simulink model "b747_lateral_openloop"  (R2025a)
settings: Solver=VariableStepAuto  StartTime=0.0  StopTime=T_end  RelTol=1e-3
undefined symbols (not defined in the file): A, B, C, D, T_end
libraries: simulink_extras x12
settings Model: Creator=User  LastModifiedBy=User

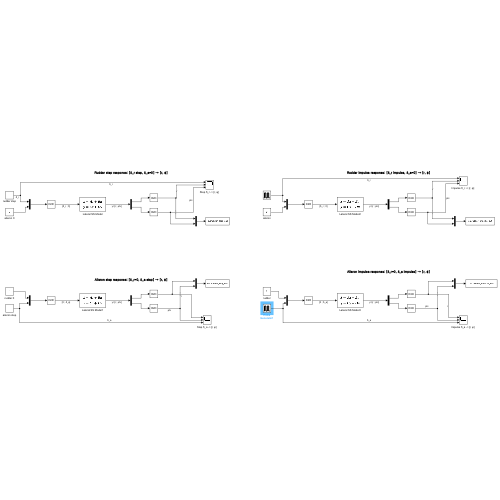
[thumbnail: Simulink's stored preview of the top-level diagram]
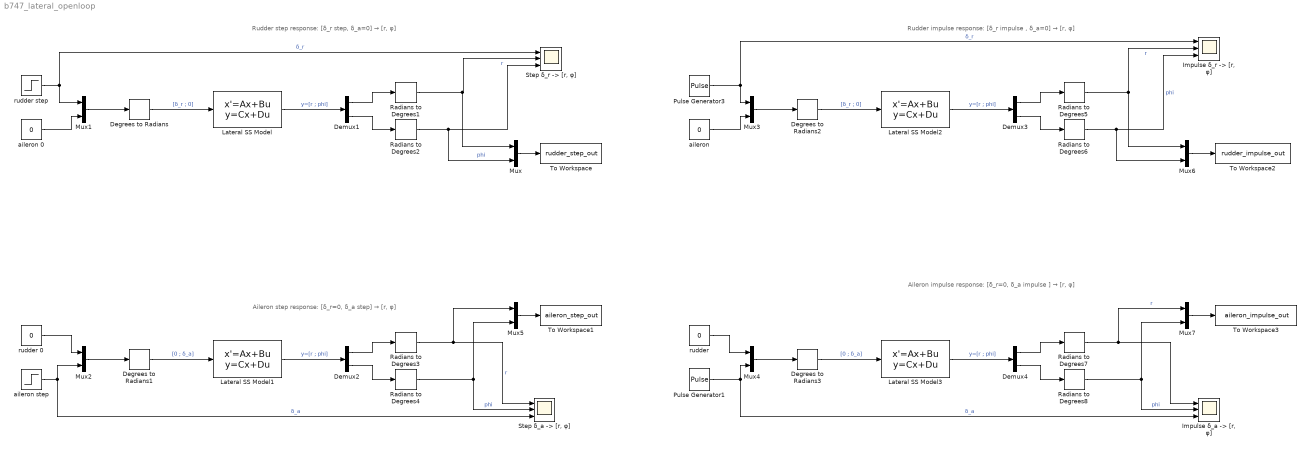
== system b747_lateral_openloop ==
  note: Rudder step response: [δ_r step, δ_a=0] → [r, φ]
  note: Aileron step response: [δ_r=0, δ_a step] → [r, φ]
  note: Aileron impulse response: [δ_r=0, δ_a impulse ] → [r, φ]
  note: Rudder impulse response: [δ_r impulse , δ_a=0] → [r, φ]
  Degrees to Radians{,1..3} (4 alike) : simulink_extras/Transformations/Degrees to Radians
  Demux{1..4} (4 alike) : Demux  Outputs=2
  "Impulse δ_a -> [r, φ] " : Scope  NumInputPorts=3
      settings: ActiveDisplayYMinimum=-7.0438793866264691  ActiveDisplayYMaximum=8.3524253239739448  DataLoggingVariableName=ScopeData6
  "Impulse δ_r -> [r, φ] " : Scope  NumInputPorts=3
      settings: ActiveDisplayYMinimum=-206.46074669660285  ActiveDisplayYMaximum=229.7370843531925  DataLoggingVariableName=ScopeData4
  Lateral SS Model{,1..3} (4 alike) : StateSpace  A=A  B=B  C=C  D=D  InitialCondition=0
  Mux{,1..7} (8 alike) : Mux  Inputs=2
  Pulse Generator1 : DiscretePulseGenerator  PulseType=Time based  Amplitude=20  Period=T_end  PulseWidth=0.125  PhaseDelay=1
  Pulse Generator3 : DiscretePulseGenerator  PulseType=Time based  Amplitude=20  Period=T_end  PulseWidth=0.125  PhaseDelay=1
  Radians to Degrees{1..8} (8 alike) : simulink_extras/Transformations/Radians to Degrees
  "Step δ_a -> [r, φ] " : Scope  NumInputPorts=3
      settings: ActiveDisplayYMinimum=-17.204068557603904  ActiveDisplayYMaximum=16.404133750150876  DataLoggingVariableName=ScopeData3
  "Step δ_r -> [r, φ] " : Scope  NumInputPorts=3
      settings: ActiveDisplayYMinimum=-259.12265026268096  ActiveDisplayYMaximum=137.01048668739392
  To Workspace : ToWorkspace  VariableName=rudder_step_out  SaveFormat=Timeseries  SampleTime=-1
  To Workspace1 : ToWorkspace  VariableName=aileron_step_out  SaveFormat=Timeseries  SampleTime=-1
  To Workspace2 : ToWorkspace  VariableName=rudder_impulse_out  SaveFormat=Timeseries  SampleTime=-1
  To Workspace3 : ToWorkspace  VariableName=aileron_impulse_out  SaveFormat=Timeseries  SampleTime=-1
  aileron : Constant  Value=0
  aileron 0 : Constant  Value=0
  aileron step : Step  SampleTime=0
  rudder : Constant  Value=0
  rudder 0 : Constant  Value=0
  rudder step : Step  SampleTime=0
  wires:
  rudder step/1 -> Mux1/1, "Step δ_r -> [r, φ] "/1  "δ_r"
  aileron 0/1 -> Mux1/2
  Degrees to Radians/1 -> Lateral SS Model/1  "[δ_r ; 0]"
  Mux1/1 -> Degrees to Radians/1
  Lateral SS Model/1 -> Demux1/1  "y=[r ; phi]"
  Demux1/1 -> Radians to Degrees1/1
  Radians to Degrees1/1 -> Mux/1, "Step δ_r -> [r, φ] "/2  "r"
  Demux1/2 -> Radians to Degrees2/1
  Lateral SS Model1/1 -> Demux2/1  "y=[r ; phi]"
  Mux2/1 -> Degrees to Radians1/1
  Radians to Degrees4/1 -> Mux5/2, "Step δ_a -> [r, φ] "/2  "phi"
  Demux2/2 -> Radians to Degrees4/1
  Degrees to Radians1/1 -> Lateral SS Model1/1  "[0 ; δ_a]"
  rudder 0/1 -> Mux2/1
  aileron step/1 -> "Step δ_a -> [r, φ] "/3, Mux2/2  "δ_a"
  Demux2/1 -> Radians to Degrees3/1
  Lateral SS Model2/1 -> Demux3/1  "y=[r ; phi]"
  Mux3/1 -> Degrees to Radians2/1
  Degrees to Radians3/1 -> Lateral SS Model3/1  "[0 ; δ_a]"
  Demux4/2 -> Radians to Degrees8/1
  Mux4/1 -> Degrees to Radians3/1
  Lateral SS Model3/1 -> Demux4/1  "y=[r ; phi]"
  Demux3/1 -> Radians to Degrees5/1
  Demux4/1 -> Radians to Degrees7/1
  Pulse Generator1/1 -> "Impulse δ_a -> [r, φ] "/3, Mux4/2  "δ_a"
  Pulse Generator3/1 -> "Impulse δ_r -> [r, φ] "/1, Mux3/1  "δ_r"
  Radians to Degrees5/1 -> "Impulse δ_r -> [r, φ] "/2, Mux6/1  "r"
  Degrees to Radians2/1 -> Lateral SS Model2/1  "[δ_r ; 0]"
  Demux3/2 -> Radians to Degrees6/1
  Radians to Degrees8/1 -> "Impulse δ_a -> [r, φ] "/2, Mux7/2  "phi"
  aileron/1 -> Mux3/2
  rudder/1 -> Mux4/1
  Radians to Degrees3/1 -> Mux5/1, "Step δ_a -> [r, φ] "/1  "r"
  Radians to Degrees2/1 -> Mux/2, "Step δ_r -> [r, φ] "/3  "phi"
  Radians to Degrees6/1 -> Mux6/2, "Impulse δ_r -> [r, φ] "/3  "phi"
  Radians to Degrees7/1 -> Mux7/1, "Impulse δ_a -> [r, φ] "/1  "r"
  Mux/1 -> To Workspace/1
  Mux5/1 -> To Workspace1/1
  Mux6/1 -> To Workspace2/1
  Mux7/1 -> To Workspace3/1
